simulink model "model_badoud"  (R2023b)
settings: Solver=FixedStepAuto  StartTime=0.0  StopTime=10  FixedStep=1e-4  RelTol=1e-5
values from neighbouring files (symbols this model uses):
  mode = 1    [25_fuzzy_inference_systeme_5.m]
  PH2 = 0    [25_fuzzy_inference_systeme_5.m]
  temp = 0    [25_fuzzy_inference_systeme_5.m]
libraries: spsPWMGeneratorDCDCLib x4, spsSeriesRLCBranchLib x3, powerlib_extras x2, spsCurrentMeasurementLib x2, spsStairGeneratorLib x2, fuzblock x1, simulink x1, slpidlib x1, spsDiodeLib x1, spsControlledVoltageSourceLib x1, spsGroundLib x1, spsIGBTLib x1
settings Model: Creator=Abdelhak_Samir  LastModifiedBy=Abdelhak_Samir
settings SolverCC: ZeroCrossAlgorithm=Adaptive
settings DebuggingCC: IgnoredZcDiagnostic=none

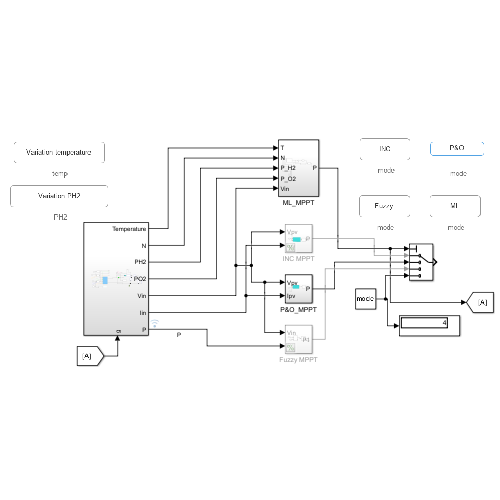
[thumbnail: Simulink's stored preview of the top-level diagram]
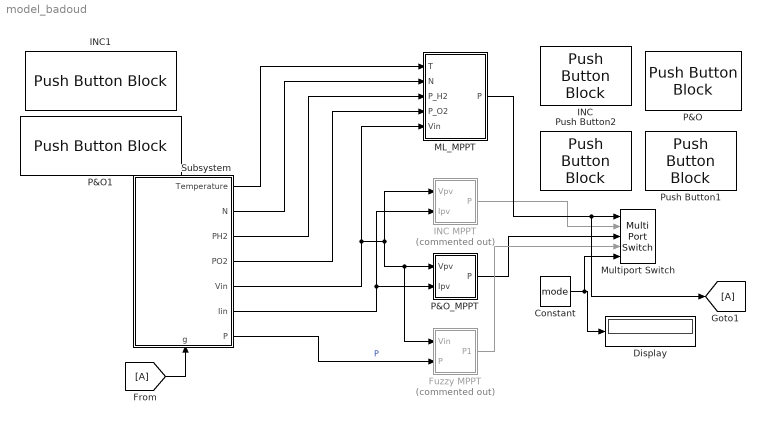
== system model_badoud ==
  Constant : Constant  Value=mode
  Display : Display
  From : From
  Fuzzy MPPT : Subsystem  Commented=on
  Goto1 : Goto
  INC : PushButtonBlock  LabelPosition=Bottom  ButtonText=INC  OnValue=2  ButtonType=Latch  OffValue=2.000000
  INC MPPT : Subsystem  Commented=on
  INC1 : PushButtonBlock  LabelPosition=Bottom  ButtonText=Variation temperature  ButtonType=Latch  OffValue=2.000000
  ML_MPPT : Subsystem
  Multiport Switch : MultiPortSwitch  Inputs=4  DiagnosticForDefault=None  SaturateOnIntegerOverflow=off  InputSameDT=off
  P&O : PushButtonBlock  LabelPosition=Bottom  ButtonText=P&O  OnValue=3  OffValue=4.000000
  P&O1 : PushButtonBlock  LabelPosition=Bottom  ButtonText=Variation PH2  OnValue=2  ButtonType=Latch  OffValue=3.000000
  P&O_MPPT : Subsystem
  Push Button1 : PushButtonBlock  LabelPosition=Bottom  ButtonText=ML  ButtonType=Latch  OffValue=4.000000
  Push Button2 : PushButtonBlock  LabelPosition=Bottom  ButtonText=Fuzzy  OnValue=4  ButtonType=Latch  OffValue=3.000000
  Subsystem : Subsystem
      settings: PortSchema="{\"entries\":[{\"content\":{\"sides\":[{\"content\":{},\"type\":\"ConnectorPlacement.EquallySpacedRectSide\",\"uuid\":\"58a8bd94-ffd4-46b6-b1a3-2be376507ce2\"},{\"content\":{\"connectorIds\":[\"Out1\",\"Out2\",\"Out3\",\"Out4\",\"Out5\",\"Out6\",\"Out7\"],\"side\":\"RIGHT\"},\"type\":\"ConnectorPlacement.EquallySpacedRectSide\",\"uuid\":\"96ef2c66-1d4c-4d1d-b7e6-2b708ee2f518\"},{\"content\":{\"side\":\"TOP\"},\"type\":\"ConnectorPlacement.EquallySpacedRectSide\",\"uuid\":\"694480ed-c70a-4162-a1ef-796d4b4241e9\"},{\"content\":{\"connectorIds\":[\"In1\"],\"side\":\"BOTTOM\"},\"type\":\"ConnectorPlacement.EquallySpacedRectSide\",\"uuid\":\"9ca02f0b-2ad8-494c-8ac8-003980ab8603\"}]},\"type\":\"ConnectorPlacement.EquallySpacedConnector\",\"uuid\":\"355acd2d-8755-4387-8227-993c4f2167fe\"}],\"packageUris\":[\"http://schema.mathworks.com/mf0/Connector/R2020b\"],\"version\":\"1.0\"}"
  wires:
  Subsystem/1(Temperature) -> ML_MPPT/1(T)
  Subsystem/2(N) -> ML_MPPT/2(N)
  Subsystem/3(PH2) -> ML_MPPT/3(P_H2)
  Subsystem/4(PO2) -> ML_MPPT/4(P_O2)
  Subsystem/5(Vin) -> Fuzzy MPPT/1(Vin), P&O_MPPT/1(Vpv), INC MPPT/1(Vpv), ML_MPPT/5(Vin)
  Subsystem/6(Iin) -> INC MPPT/2(Ipv), P&O_MPPT/2(Ipv)
  Subsystem/7(P) -> Fuzzy MPPT/2(P)  "P"
  Constant/1 -> Multiport Switch/5, Display/1
  From/1 -> Subsystem/1(g)
  INC MPPT/1(P) -> Multiport Switch/2
  P&O_MPPT/1(P) -> Multiport Switch/3
  Fuzzy MPPT/1(P1) -> Multiport Switch/4
  ML_MPPT/1(P) -> Goto1/1, Multiport Switch/1

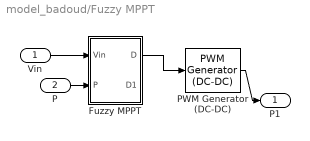
== system model_badoud/Fuzzy MPPT ==
  Vin : Inport
  P : Inport  Port=2
  Fuzzy MPPT : Subsystem
  PWM Generator (DC-DC) : spsPWMGeneratorDCDCLib/PWM Generator (DC-DC)  Fsw=20e2  Ts=1e-4
  P1 : Outport
  wires:
  Vin/1 -> Fuzzy MPPT/1(Vin)
  Fuzzy MPPT/1(D) -> PWM Generator (DC-DC)/1
  P/1 -> Fuzzy MPPT/2(P)
  PWM Generator (DC-DC)/1 -> P1/1

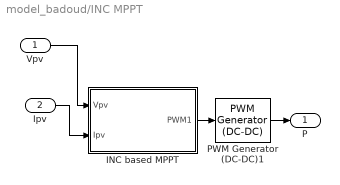
== system model_badoud/INC MPPT ==
  Vpv : Inport
  Ipv : Inport  Port=2
  INC based MPPT : Subsystem
  PWM Generator (DC-DC)1 : spsPWMGeneratorDCDCLib/PWM Generator (DC-DC)  Fsw=20e2  Ts=1e-4
  P : Outport
  wires:
  INC based MPPT/1(PWM1) -> PWM Generator (DC-DC)1/1
  Vpv/1 -> INC based MPPT/1(Vpv)
  Ipv/1 -> INC based MPPT/2(Ipv)
  PWM Generator (DC-DC)1/1 -> P/1

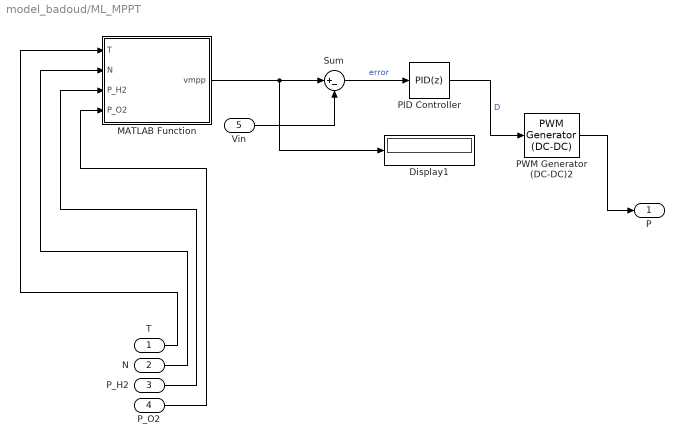
== system model_badoud/ML_MPPT ==
  T : Inport
  N : Inport  Port=2
  P_H2 : Inport  Port=3
  P_O2 : Inport  Port=4
  Vin : Inport  Port=5
  Display1 : Display
  MATLAB Function : MATLAB Function  TreatAsAtomicUnit=on
  PID Controller : slpidlib/PID Controller  Controller=PID  Form=Parallel  TimeDomain=Discrete-time  UseExternalTs=off  SampleTime=1e-4  IntegratorMethod=Forward Euler  FilterMethod=Forward Euler  ControllerParametersSource=internal  P=-10.122  I=-0.00125  UseKiTs=off  D=0.014  N=0  UseFilter=on  TunerSelectOption=Frequency Response Based  InitialConditionSource=internal  InitialConditionForIntegrator=0  InitialConditionForFilter=0  DifferentiatorICPrevScaledInput=0  ExternalReset=none  TrackingMode=off  Kt=1  LimitOutput=off  SatLimitsSource=internal  UpperSaturationLimit=inf  LowerSaturationLimit=-inf  LinearizeAsGain=on  AntiWindupMode=none  Kb=1  LimitIntegrator=off  UpperIntegratorSaturationLimit=inf  LowerIntegratorSaturationLimit=-inf  POutMin=[]  POutMax=[]  IOutMin=[]  IOutMax=[]  DOutMin=[]  DOutMax=[]  NOutMin=[]  NOutMax=[]  SumOutMin=[]  SumOutMax=[]  SaturationOutMin=[]  SaturationOutMax=[]  PParamMin=[]  PParamMax=[]  IParamMin=[]  IParamMax=[]  DParamMin=[]  DParamMax=[]  NParamMin=[]  NParamMax=[]  KbParamMin=[]  KbParamMax=[]  KtParamMin=[]  KtParamMax=[]  KbOutMin=[]  KbOutMax=[]  KtOutMin=[]  KtOutMax=[]  IntegratorOutMin=[]  IntegratorOutMax=[]  FilterOutMin=[]  FilterOutMax=[]  SumI1OutMin=[]  SumI1OutMax=[]  SumI2OutMin=[]  SumI2OutMax=[]  SumI3OutMin=[]  SumI3OutMax=[]  SumI4OutMin=[]  SumI4OutMax=[]  SumDOutMin=[]  SumDOutMax=[]  DifferentiatorOutMin=[]  DifferentiatorOutMax=[]  FilterDiffOutCoefMin=[]  FilterDiffOutCoefMax=[]  ReciprocalOutMin=[]  ReciprocalOutMax=[]  SumDenOutMin=[]  SumDenOutMax=[]  SumNumOutMin=[]  SumNumOutMax=[]  DivideOutMin=[]  DivideOutMax=[]  UdiffTsProdOutMin=[]  UdiffTsProdOutMax=[]  NTsProdOutMin=[]  NTsProdOutMax=[]  UintegralTsProdOutMin=[]  UintegralTsProdOutMax=[]  UngainTsProdOutMin=[]  UngainTsProdOutMax=[]  ClampingZeroOutDataTypeStr=Inherit: Inherit via back propagation  ClampingZeroOutMin=[]  ClampingZeroOutMax=[]  FilterDenConstantOutDataTypeStr=Inherit: Inherit via back propagation  FilterDenConstantOutMin=[]  FilterDenConstantOutMax=[]  PCopyOutDataTypeStr=Inherit: Inherit via back propagation  PCopyOutMin=[]  PCopyOutMax=[]  NCopyOutDataTypeStr=Inherit: Inherit via back propagation  NCopyOutMin=[]  NCopyOutMax=[]  IntegratorContinuousStateAttributes=''  IntegratorStateMustResolveToSignalObject=off  IntegratorRTWStateStorageClass=Auto  FilterContinuousStateAttributes=''  FilterStateMustResolveToSignalObject=off  FilterRTWStateStorageClass=Auto  ParallelPVariant=InternalParameters  IdealPVariant=Disabled  IVariant=InternalParameters  DVariant=InternalParameters  IntegratorVariant=Discrete  SatVariant=Disabled  AWVariant=Passthrough  PCopyVariant=Disabled  TRVariant=Disabled  FdbkBlocksVariant=Forward  IdealPFdbkVariant=Disabled  SatFdbkVariant=Disabled  DerivativeFilterVariant=ForwardEulerFilter  NVariant=InternalParameters  NCopyVariant=Disabled  FilterICVariant=InternalICsFilter  IntegratorICVariant=InternalICs  ExternalResetVariant=Disabled  TRSumVariant=Passthrough  SumFdbkVariant=Disabled  SumVariant=Sum_PID  TsampFilterVariant=InternalTs  TsampNgainVariant=Passthrough  TsampIntegralVariant=Disabled_SignalSpec  ExternalSaturationOutDataTypeStr=Inherit: Same as second input
  PWM Generator (DC-DC)2 : spsPWMGeneratorDCDCLib/PWM Generator (DC-DC)  Fsw=20e2  Ts=1e-4
  Sum : Sum  Inputs=|+-
  P : Outport
  wires:
  MATLAB Function/1(vmpp) -> Display1/1, Sum/1
  P_H2/1 -> MATLAB Function/3(P_H2)
  Sum/1 -> PID Controller/1  "error"
  PID Controller/1 -> PWM Generator (DC-DC)2/1  "D"
  Vin/1 -> Sum/2
  PWM Generator (DC-DC)2/1 -> P/1
  T/1 -> MATLAB Function/1(T)
  N/1 -> MATLAB Function/2(N)
  P_O2/1 -> MATLAB Function/4(P_O2)

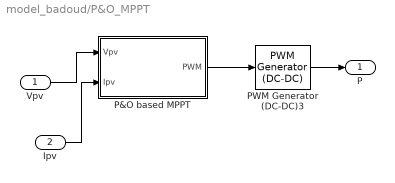
== system model_badoud/P&O_MPPT ==
  Vpv : Inport
  Ipv : Inport  Port=2
  P&O based MPPT : Subsystem
  PWM Generator (DC-DC)3 : spsPWMGeneratorDCDCLib/PWM Generator (DC-DC)  Fsw=20e2  Ts=1e-4
  P : Outport
  wires:
  P&O based MPPT/1(PWM) -> PWM Generator (DC-DC)3/1
  Vpv/1 -> P&O based MPPT/1(Vpv)
  PWM Generator (DC-DC)3/1 -> P/1
  Ipv/1 -> P&O based MPPT/2(Ipv)

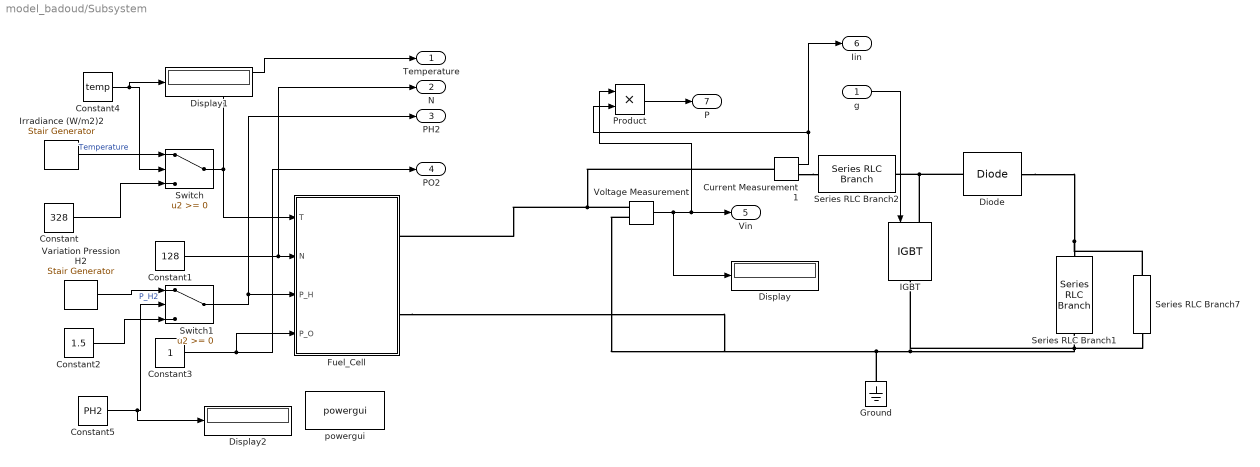
== system model_badoud/Subsystem ==
  g : Inport
  Constant : Constant  Value=328
  Constant1 : Constant  Value=128
  Constant2 : Constant  Value=1.5
  Constant3 : Constant
  Constant4 : Constant  Value=temp
  Constant5 : Constant  Value=PH2
  Current Measurement1 : spsCurrentMeasurementLib/Current Measurement  PhasorSimulation=off  OutputType=Complex  PSBequivalent=0
  Diode : spsDiodeLib/Diode  Ron=0.001  Lon=0  Vf=0.8  IC=0  UseSnubber=0  Rs=500  Cs=250e-9  Measurements=off
  Display : Display
  Display1 : Display
  Display2 : Display
  Fuel_Cell : Subsystem
  Ground : spsGroundLib/Ground  LConnTagsString=a
  IGBT : spsIGBTLib/IGBT  Ron=0.001  Lon=0  Vf=1  Tf=1e-6  Tt=2e-6  IC=0  Rs=1e5  Cs=inf  Measurements=off
  Irradiance (W/m2)2 : spsStairGeneratorLib/Stair Generator  t=[0, 0.2 , 0.4 , 0.6, 0.8, 1]  e=[300,320,330,310,300,330]  Ts=1e-4
  Product : Product
  Series RLC Branch1 : spsSeriesRLCBranchLib/Series RLC Branch  LConnTagsString=__new0  RConnTagsString=__new0  BranchType=C  Resistance=0.1  Inductance=1e-3  SetiL0=off  InitialCurrent=0  Capacitance=1e-6  Setx0=off  InitialVoltage=0  Measurements=None
  Series RLC Branch2 : spsSeriesRLCBranchLib/Series RLC Branch  LConnTagsString=__new0  RConnTagsString=__new0  BranchType=L  Resistance=0.1  Inductance=0.98  SetiL0=off  InitialCurrent=0  Capacitance=1e-6  Setx0=off  InitialVoltage=0  Measurements=None
  Series RLC Branch7 : spsSeriesRLCBranchLib/Series RLC Branch  LConnTagsString=__new0  RConnTagsString=__new0  BranchType=R  Resistance=26  Inductance=1e-3  SetiL0=off  InitialCurrent=0  Capacitance=400e-6  Setx0=off  InitialVoltage=0  Measurements=None
  Switch : Switch  SaturateOnIntegerOverflow=off  InputSameDT=off
  Switch1 : Switch  SaturateOnIntegerOverflow=off  InputSameDT=off
  Variation Pression H2 : spsStairGeneratorLib/Stair Generator  t=[0, 0.2 , 0.4 , 0.6, 0.8, 1]  e=[1,1.5,0.5,1,0.5,1.5]  Ts=1e-4
  Voltage Measurement : spsVoltageMeasurementLib/Voltage Measurement  PhasorSimulation=off  OutputType=Complex  PSBequivalent=0
  powergui : spspowerguiLib/powergui  Priority=1  SimulationMode=Discrete  SampleTime=1e-4  frequency=60  Iterations=50  frequencyindice=0  Pbase=100e6  ErrMax=1e-4  UnitsV=kV  UnitsW=MW  buscounter=0  FunctionMessages=off  echomessages=off  EnableUseOfTLC=off  CurrentSourceSwitches=off  DisableSnubberDevices=off  DisableRonSwitches=off  DisableVfSwitches=off  DisplayEquations=off  AutomaticDiscreteSolvers=off  SolverType=Tustin/Backward Euler (TBE)  Interpol=off  ExternalGateDelay=off  methode=off  Ts=100  x0status=blocks  SPID=on  SwTol=0  HookPort=off  NonlinearTolerance=1e-4  nMaxIteration=100  ContinueOnMaxIteration=off  RestoreLinks=warning  ResistiveCurrentMeasurement=off  Frange=[0:2:500]  Ylog=off  Xlog=on  ShowGrid=off  save=off  variable=ZData  structure=0  ZoomFFT=off  StartTime=0.0  cycles=1  DisplayStyle=1  fundamental=60  FreqAxis=off  MaxFrequency=1000  frequencyindicesteady=1  RmsSteady=1  display=off
  Temperature : Outport
  N : Outport  Port=2
  PH2 : Outport  Port=3
  PO2 : Outport  Port=4
  Vin : Outport  Port=5
  Iin : Outport  Port=6
  P : Outport  Port=7
  wires:
  Constant1/1 -> N/1, Fuel_Cell/2(N)
  Constant3/1 -> PO2/1, Fuel_Cell/4(P_O)
  Product/1 -> P/1
  Voltage Measurement/1 -> Product/1, Vin/1, Display/1
  Current Measurement1/1 -> Iin/1, Product/2
  g/1 -> IGBT/1
  Switch/1 -> Temperature/1, Fuel_Cell/1(T)
  Irradiance (W/m2)2/1 -> Switch/1  "Temperature"
  Constant/1 -> Switch/3
  Constant4/1 -> Display1/1, Switch/2
  Switch1/1 -> Fuel_Cell/3(P_H), PH2/1
  Variation Pression H2/1 -> Switch1/1  "P_H2"
  Constant2/1 -> Switch1/3
  Constant5/1 -> Display2/1, Switch1/2
  connections:
  Ground/LConn1 -- Voltage Measurement/LConn2 -- Fuel_Cell/RConn2 -- IGBT/RConn1 -- Series RLC Branch1/RConn1 -- Series RLC Branch7/RConn1
  IGBT/LConn1 -- Diode/LConn1 -- Series RLC Branch2/RConn1
  Series RLC Branch1/LConn1 -- Diode/RConn1 -- Series RLC Branch7/LConn1
  Current Measurement1/RConn1 -- Series RLC Branch2/LConn1
  Voltage Measurement/LConn1 -- Current Measurement1/LConn1 -- Fuel_Cell/RConn1

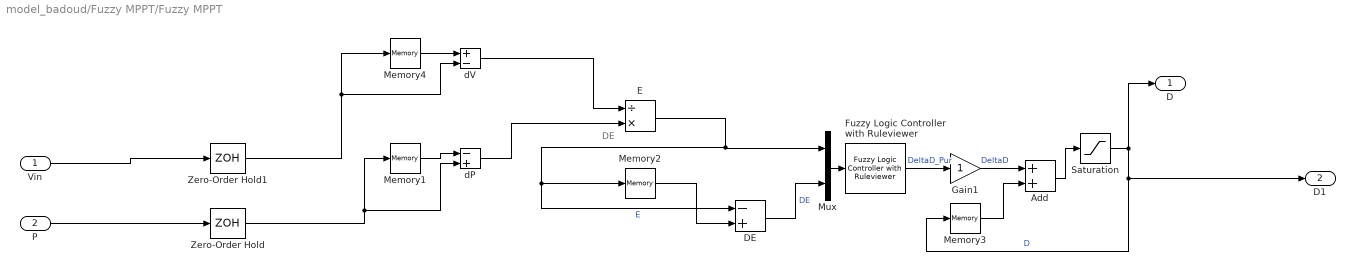
== system model_badoud/Fuzzy MPPT/Fuzzy MPPT ==
  note: DE
  Vin : Inport
  P : Inport  Port=2
  Add : Sum
  DE : Sum  Inputs=-+
  E : Product  Inputs=/*
  Fuzzy Logic Controller with Ruleviewer : fuzblock/Fuzzy Logic  Controller  with Ruleviewer  fismatrix=twnty_five_rules_5  Ts=1
  Gain1 : Gain
  Memory1 : Memory  InheritSampleTime=on
  Memory2 : Memory  InheritSampleTime=on
  Memory3 : Memory
  Memory4 : Memory  InheritSampleTime=on
  Mux : Mux  Inputs=2
  Saturation : Saturate  UpperLimit=0.9  LowerLimit=0.1
  Zero-Order Hold : ZeroOrderHold  SampleTime=-1
  Zero-Order Hold1 : ZeroOrderHold  SampleTime=-1
  dP : Sum  Inputs=-+
  dV : Sum  Inputs=+-
  D : Outport
  D1 : Outport  Port=2
  wires:
  DE/1 -> Mux/2  "DE"
  Fuzzy Logic Controller with Ruleviewer/1 -> Gain1/1  "DeltaD_Pur"
  Zero-Order Hold/1 -> dP/2, Memory1/1
  dV/1 -> E/1
  dP/1 -> E/2
  E/1 -> DE/1, Memory2/1, Mux/1  "E"
  Mux/1 -> Fuzzy Logic Controller with Ruleviewer/1
  Memory4/1 -> dV/1
  Memory1/1 -> dP/1
  Zero-Order Hold1/1 -> Memory4/1, dV/2
  Gain1/1 -> Add/1  "DeltaD"
  Memory3/1 -> Add/2
  Saturation/1 -> D/1, D1/1, Memory3/1  "D"
  Memory2/1 -> DE/2
  Add/1 -> Saturation/1
  Vin/1 -> Zero-Order Hold1/1
  P/1 -> Zero-Order Hold/1

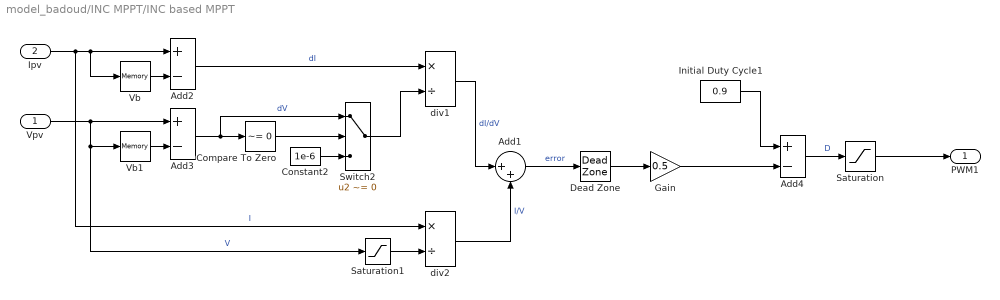
== system model_badoud/INC MPPT/INC based MPPT ==
  Vpv : Inport
  Ipv : Inport  Port=2
  Add1 : Sum  Inputs=|++
  Add2 : Sum  Inputs=+-
  Add3 : Sum  Inputs=+-
  Add4 : Sum  Inputs=+-
  Compare To Zero : simulink/Logic and Bit Operations/Compare To Zero  relop=~=  OutDataTypeStr=uint8
  Constant2 : Constant  Value=1e-6
  Dead Zone : DeadZone  LowerValue=-0.02  UpperValue=+0.02
  Gain : Gain  Gain=0.5
  Initial Duty Cycle1 : Constant  Value=0.9
  Saturation : Saturate  UpperLimit=0.9  LowerLimit=0.1
  Saturation1 : Saturate  UpperLimit=inf  LowerLimit=eps
  Switch2 : Switch  Criteria=u2 ~= 0  SaturateOnIntegerOverflow=off  InputSameDT=off
  Vb : Memory  InheritSampleTime=on  LinearizeAsDelay=on
  Vb1 : Memory  InheritSampleTime=on  LinearizeAsDelay=on
  div1 : Product  Inputs=*/  RndMeth=Zero
  div2 : Product  Inputs=*/  RndMeth=Zero
  PWM1 : Outport
  wires:
  Add4/1 -> Saturation/1  "D"
  Gain/1 -> Add4/2
  Initial Duty Cycle1/1 -> Add4/1
  Add3/1 -> Compare To Zero/1, Switch2/1  "dV"
  div2/1 -> Add1/2  "I/V"
  Saturation1/1 -> div2/2
  Vb1/1 -> Add3/2
  Add2/1 -> div1/1  "dI"
  Switch2/1 -> div1/2
  Vb/1 -> Add2/2
  Ipv/1 -> Vb/1, Add2/1, div2/1  "I"
  div1/1 -> Add1/1  "dI/dV"
  Compare To Zero/1 -> Switch2/2
  Constant2/1 -> Switch2/3
  Vpv/1 -> Add3/1, Vb1/1, Saturation1/1  "V"
  Add1/1 -> Dead Zone/1  "error"
  Dead Zone/1 -> Gain/1
  Saturation/1 -> PWM1/1

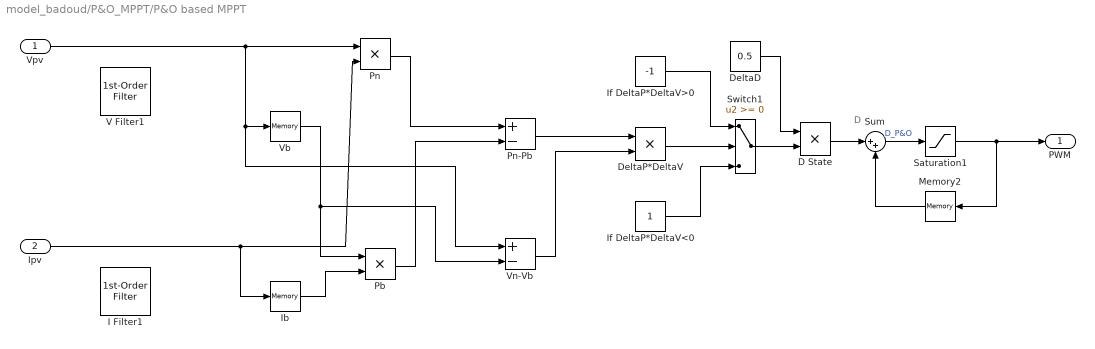
== system model_badoud/P&O_MPPT/P&O based MPPT ==
  note: D
  Vpv : Inport
  Ipv : Inport  Port=2
  D State : Product  RndMeth=Zero
  DeltaD : Constant  Value=0.5
  DeltaP*DeltaV : Product  RndMeth=Zero
  I Filter1 : powerlib_extras/Control  Blocks/1st-Order  Filter  FilterType=Lowpass  Tc=1e-3  Initialize=off  Vac_Init=[0.8 -25 60]  Vdc_Init=-0.4  PlotResponse=off  param1=[1 500 1]
  Ib : Memory  InheritSampleTime=on  LinearizeAsDelay=on
  If DeltaP*DeltaV<0 : Constant
  If DeltaP*DeltaV>0 : Constant  Value=-1
  Memory2 : Memory  InheritSampleTime=on
  Pb : Product  RndMeth=Zero
  Pn : Product  RndMeth=Zero
  Pn-Pb : Sum  Inputs=+-
  Saturation1 : Saturate  UpperLimit=0.9  LowerLimit=0.1
  Sum : Sum  Inputs=|++
  Switch1 : Switch  SaturateOnIntegerOverflow=off  InputSameDT=off
  V Filter1 : powerlib_extras/Control  Blocks/1st-Order  Filter  FilterType=Lowpass  Tc=1e-3  Initialize=off  Vac_Init=[0.8 -25 60]  Vdc_Init=-0.4  PlotResponse=off  param1=[1 500 1]
  Vb : Memory  InheritSampleTime=on  LinearizeAsDelay=on
  Vn-Vb : Sum  Inputs=+-
  PWM : Outport
  wires:
  If DeltaP*DeltaV<0/1 -> Switch1/3
  Pn/1 -> Pn-Pb/1
  Vpv/1 -> Vn-Vb/1, Vb/1, Pn/1
  Ib/1 -> Pb/2
  DeltaP*DeltaV/1 -> Switch1/2
  Vb/1 -> Vn-Vb/2, Pb/1
  If DeltaP*DeltaV>0/1 -> Switch1/1
  Pn-Pb/1 -> DeltaP*DeltaV/1
  Vn-Vb/1 -> DeltaP*DeltaV/2
  Ipv/1 -> Pn/2, Ib/1
  Pb/1 -> Pn-Pb/2
  Switch1/1 -> D State/2
  DeltaD/1 -> D State/1
  D State/1 -> Sum/1
  Sum/1 -> Saturation1/1  "D_P&O"
  Memory2/1 -> Sum/2
  Saturation1/1 -> PWM/1, Memory2/1

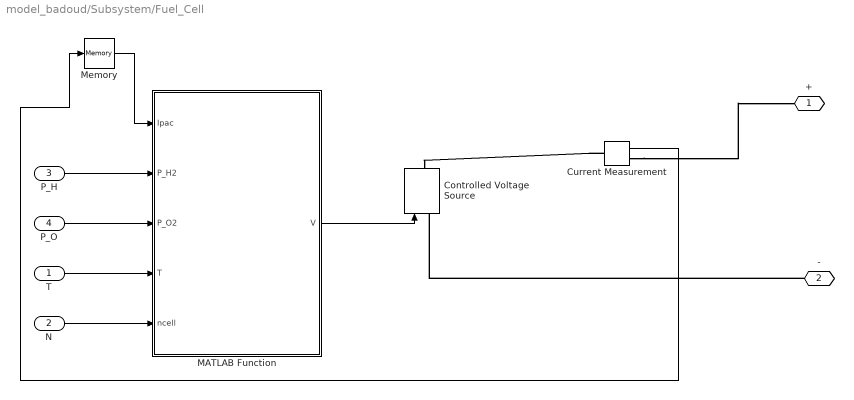
== system model_badoud/Subsystem/Fuel_Cell ==
  T : Inport
  N : Inport  Port=2
  P_H : Inport  Port=3
  P_O : Inport  Port=4
  Controlled Voltage Source : spsControlledVoltageSourceLib/Controlled Voltage Source  Initialize=on  Source_Type=AC  Amplitude=0  Phase=0  Frequency=0  Measurements=None
  Current Measurement : spsCurrentMeasurementLib/Current Measurement  PhasorSimulation=off  OutputType=Complex  PSBequivalent=0
  MATLAB Function : MATLAB Function  TreatAsAtomicUnit=on
  Memory : Memory  InitialCondition=1e-4  InheritSampleTime=on
  + : PMIOPort  Side=Right
  - : PMIOPort  Port=2  Side=Right
  wires:
  P_H/1 -> MATLAB Function/2(P_H2)
  P_O/1 -> MATLAB Function/3(P_O2)
  N/1 -> MATLAB Function/5(ncell)
  T/1 -> MATLAB Function/4(T)
  MATLAB Function/1(V) -> Controlled Voltage Source/1
  Current Measurement/1 -> Memory/1
  Memory/1 -> MATLAB Function/1(Ipac)
  connections:
  Current Measurement/LConn1 -- Controlled Voltage Source/RConn1
  Current Measurement/RConn1 -- +/RConn1
  -/RConn1 -- Controlled Voltage Source/LConn1

== matlab function model_badoud/Subsystem/Fuel_Cell/MATLAB Function ==
  data: Ipac input; V output; P_H2 input; P_O2 input; T input; ncell input
function V  =Fuel_Cell(Ipac,P_H2,P_O2,T,ncell) 
%% l'equation de nernest :
A=70;% la surface active de la pile 
x1=P_H2;
x2=P_O2;
Enernst=1.229-(0.85e-3)*(T-298.15)+(4.31e-5*T*(ln(P_H2)-0.5*ln(P_O2)));
%% voltage d'activation :
 C_H2=P_H2/(1.1*10.^(6)* exp(-77/T));
x3=C_H2;
C_O2= P_O2/(5.08.*10.^(5).*exp((-498)/T));
x4=C_O2;
k1=-0.514;
x7=A;
% k2= 0.00286+(0.0002*ln(A))+(4.3ln*(CH2)*10.^(5));
k2=0.00286 + 0.0002*ln(A)+(4.3*ln(C_H2)*10.^(-5));
k3=0.41e-4;
k4=-0.93e-4;
x5=Ipac;
Vact=-(k1+(k2*T)+(k3*T*ln(x4))+(k4*T*ln(x5)));

%% le voltage homique :
R_C=15e-4;%la resistance equivalente de contact a la conduction des electrons : 
Y=27.7;% teneur de l'eau dans la membrane
% la résistance spécifique de la membrane :
r_M=181.6*(1+(0.03*(Ipac/A))+(0.062*((T/303).^(2))*((Ipac/A).^(2.5)))/((Y-0.634-(3*(Ipac/A)))*exp(4.18*(T-303)/T)));
R_M=0.0128*r_M/A;
Vomh=Ipac*(R_M+R_C);
%%  le voltage de concentration :
B=0.0016;
Jmax=1.5;% densite de courant max 
J=Ipac/A;
x6=1-(J/Jmax);
Vconc=-B*ln(x6); 
%% le voltage  d'une cellule  :
U=Enernst-Vact-Vomh-Vconc;
%%  le  voltages  total :
V=ncell*U;

== matlab function model_badoud/ML_MPPT/MATLAB Function ==
  data: T input; N input; vmpp output; P_H2 input; P_O2 input
function vmpp = fcn(T, N,P_H2, P_O2)
    vmpp = N*(predict_vmpp_matlab_model(T, P_H2, P_O2) - 0.703125);
end
